simulink model "FOC"  (R2017a)
settings: Solver=VariableStepAuto  StartTime=0.0  StopTime=2.5  MaxStep=1e-4  RelTol=1e-3  EnableMultiTasking=on
values from neighbouring files (symbols this model uses):
  Ki_i = Tc/(2*Kc*Tsum)    (= 11.475)    [FOC_parameters.m]
  Ki_n = Kp_n/Ti_n    (= 1)    [FOC_parameters.m]
  Kp_i = Ki_i*Ti_i    (= 0.017)    [FOC_parameters.m]
  Kp_n = 1    [FOC_parameters.m]
  Ld = 8.5e-3    (= 0.0085)    [FOC_parameters.m]
  Lq = Ld    (= 0.0085)    [FOC_parameters.m]
  m = 1    [FOC_parameters.m]
  n_s = 1    [FOC_parameters.m]
  p = 4    [FOC_parameters.m]
  Rs = 0.0485    [FOC_parameters.m]
  Tf = 0    [FOC_parameters.m]
  Ti = 0.0027    [FOC_parameters.m]
  TL = 400    [FOC_parameters.m]
  vd = 0.0004924    [FOC_parameters.m]
libraries: powerlib x4, powerlib_meascontrol x2
settings Model: Creator=Noxma  LastModifiedBy=s181835
settings OptimizationCC: LifeSpan=inf
settings DebuggingCC: SFUnexpectedBacktrackingDiag=warning  SFNoUnconditionalDefaultTransitionDiag=warning  SFExecutionAtInitializationDiag=none
settings GRTTargetCC: TargetLangStandard=C89/C90 (ANSI)  GeneratePreprocessorConditionals=Disable all
settings ConfigComp: CovMetricSettings=dw  CovHtmlReporting=on  CovSaveCumulativeToWorkspaceVar=on  CovSaveSingleToWorkspaceVar=on  CovExternalEMLEnable=off

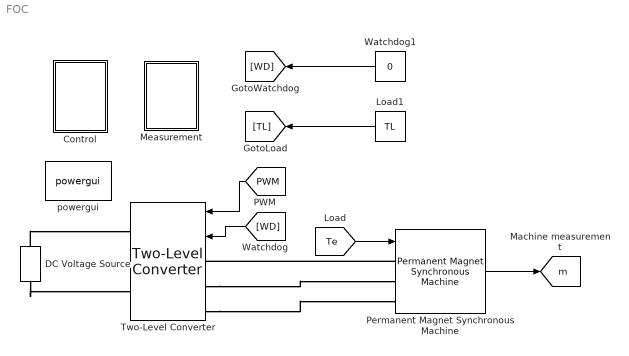
== system FOC ==
  Control : Subsystem
  DC Voltage Source : powerlib/Electrical Sources/DC Voltage Source  Amplitude=1  Measurements=None
  Load1 : Constant  Value=TL
  Measurement : Subsystem
  Permanent Magnet Synchronous Machine : powerlib/Machines/Permanent Magnet Synchronous Machine  NbPhases=3  FluxDistribution=Sinusoidal  RotorType=Salient-pole  MechanicalLoad=Torque Tm  PresetModel=No  ShowDetailedParameters=on  MeasurementBus=on  Resistance=Rs  Inductance=8.5e-3  dqInductances=[Ld,Lq]  La=0.000395  MachineConstant=Flux linkage established by magnets (V.s)  Flux=cphi  VoltageCst=86.6271  TorqueCst=0.7164  Flat=120  Mechanical=[Ti vd p Tf]  PolePairs=4  InitialConditions=[0,0, 0,0]  InitialConditions5ph=[0 0 0 0 0 0]  TsPowergui=0  TsBlock=-1  RefAngle=90 degrees behind phase A axis (modified Park)
      settings: SourceProductName=Simscape Power Systems
  Two-Level Converter : powerlib/Power Electronics/Two-Level Converter  ModelType=Switching devices  Ron=1e-3  Rs=1e6  Cs=inf  Vforward=[0,0]  Ron_Diode=1e-3  Rs_Diode=1e6  Cs_Diode=inf  Vf_Diode=1e-3  Rs_CurrentSource=inf
      settings: SourceProductName=Simscape Power Systems  SourceProductBaseCode=PS
  Watchdog1 : Constant  Value=0
  powergui : powerlib/powergui  Priority=1  SimulationMode=Continuous  SampleTime=50e-6  frequency=60  Iterations=50  frequencyindice=0  Pbase=100e6  ErrMax=1e-4  UnitsV=kV  UnitsW=MW  buscounter=0  FunctionMessages=off  echomessages=off  EnableUseOfTLC=off  CurrentSourceSwitches=off  DisableSnubberDevices=off  DisableRonSwitches=off  DisableVfSwitches=off  DisplayEquations=off  SolverType=Tustin/Backward Euler (TBE)  Interpol=off  ExternalGateDelay=off  methode=off  Ts=100  x0status=blocks  SPID=on  SwTol=0  HookPort=off  RestoreLinks=warning  ResistiveCurrentMeasurement=off  Frange=[0:2:500]  Ylog=off  Xlog=on  ShowGrid=off  save=off  variable=ZData  structure=0  ZoomFFT=off  StartTime=0.0  cycles=1  DisplayStyle=1  fundamental=60  FreqAxis=off  MaxFrequency=1000  frequencyindicesteady=1  RmsSteady=1  display=off
  tag scope: m=global
  wires:
  [PWM] -> Two-Level Converter/1
  [Te] -> Permanent Magnet Synchronous Machine/1
  Permanent Magnet Synchronous Machine/1 -> [m]
  [WD] -> Two-Level Converter/2
  Watchdog1/1 -> [WD]
  Load1/1 -> [TL]
  connections:
  Two-Level Converter/LConn3 -- Permanent Magnet Synchronous Machine/LConn3
  Two-Level Converter/LConn2 -- Permanent Magnet Synchronous Machine/LConn2
  Permanent Magnet Synchronous Machine/LConn1 -- Two-Level Converter/LConn1
  DC Voltage Source/LConn1 -- Two-Level Converter/RConn2
  DC Voltage Source/RConn1 -- Two-Level Converter/RConn1

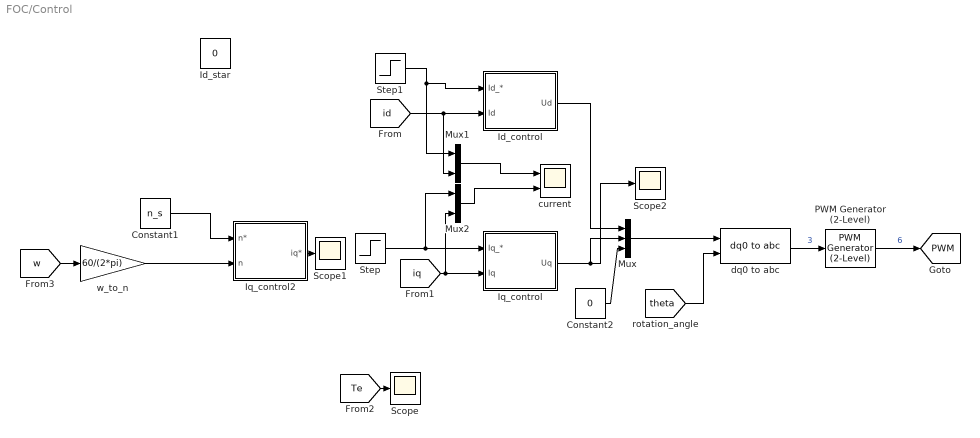
== system FOC/Control ==
  Constant1 : Constant  Value=n_s
  Constant2 : Constant  Value=0
  Id_control : Subsystem
  Id_star : Constant  Value=0
  Iq_control : Subsystem
  Iq_control2 : Subsystem
  Mux : Mux  Inputs=3
  Mux1 : Mux  Inputs=2
  Mux2 : Mux  Inputs=2
  PWM Generator (2-Level) : powerlib_meascontrol/Pulse & Signal Generators/PWM Generator (2-Level)  ModulatorType=Three-phase bridge (6 pulses)  ModulatorMode=Unsynchronized  Fc=fs  Pc=pwm_angle  nF=27  MinMax=[-m m]  SamplingTechnique=Natural  ModulatingSignals=off  m=1  Freq=f  Phase=0  Ts=0  ShowCarrierOutport=off
      settings: SourceProductName=Simscape Power Systems
  Scope : Scope
  Scope1 : Scope
  Scope2 : Scope
  Step : Step  Time=0.2  After=3  SampleTime=0
  Step1 : Step  Time=1.5  After=-1  SampleTime=0
  current : Scope  NumInputPorts=2
  dq0 to abc : powerlib_meascontrol/Transformations/dq0 to abc  Alignment=90 degrees behind phase A axis
  w_to_n : Gain  Gain=60/(2*pi)
  tag scope: PWM=global
  wires:
  PWM Generator (2-Level)/1 -> [PWM]  "6"
  [id] -> Mux1/2, Id_control/2(Id)
  [iq] -> Iq_control/2(Iq), Mux2/2
  Iq_control/1(Uq) -> Scope2/1, Mux/2
  Id_control/1(Ud) -> Mux/1
  Mux/1 -> dq0 to abc/1
  [theta] -> dq0 to abc/2
  [w] -> w_to_n/1
  w_to_n/1 -> Iq_control2/2(n)
  Constant1/1 -> Iq_control2/1(n*)
  [Te] -> Scope/1
  Constant2/1 -> Mux/3
  Step/1 -> Mux2/1, Iq_control/1(Iq_*)
  dq0 to abc/1 -> PWM Generator (2-Level)/1  "3"
  Iq_control2/1(iq*) -> Scope1/1
  Mux1/1 -> current/1
  Mux2/1 -> current/2
  Step1/1 -> Id_control/1(Id_*), Mux1/1

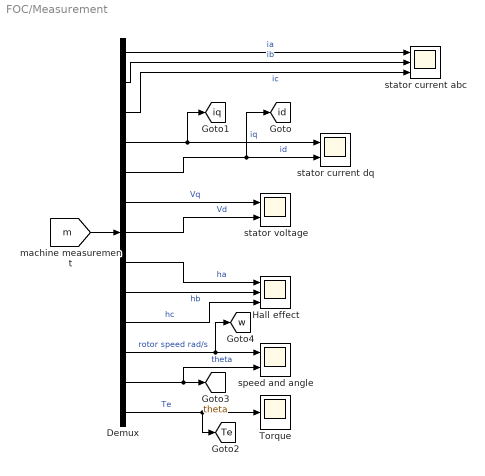
== system FOC/Measurement ==
  Demux : Demux  Outputs=13
  Hall effect : Scope  NumInputPorts=3
  Torque : Scope
  speed and angle : Scope  NumInputPorts=2
  stator current abc : Scope  NumInputPorts=3
  stator current dq : Scope  NumInputPorts=2
  stator voltage : Scope  NumInputPorts=2
  tag scope: Te=global, id=global, iq=global, theta=global, w=global
  wires:
  Demux/5 -> [id], stator current dq/2  "id"
  Demux/2 -> stator current abc/2  "ib"
  Demux/4 -> [iq], stator current dq/1  "iq"
  Demux/13 -> [Te], Torque/1  "Te"
  [m] -> Demux/1
  Demux/9 -> Hall effect/2  "hb"
  Demux/6 -> stator voltage/1  "Vq"
  Demux/11 -> [w], speed and angle/1  "rotor speed rad/s"
  Demux/12 -> [theta], speed and angle/2  "theta"
  Demux/7 -> stator voltage/2  "Vd"
  Demux/8 -> Hall effect/1  "ha"
  Demux/10 -> Hall effect/3  "hc"
  Demux/3 -> stator current abc/3  "ic"
  Demux/1 -> stator current abc/1  "ia"

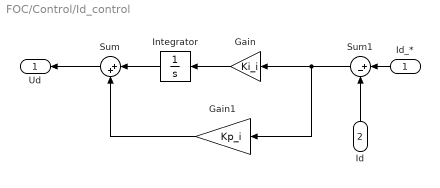
== system FOC/Control/Id_control ==
  Id_* : Inport
  Id : Inport  Port=2
  Gain : Gain  Gain=Ki_i
  Gain1 : Gain  Gain=Kp_i
  Integrator : Integrator
  Sum : Sum  Inputs=|++
  Sum1 : Sum  Inputs=|+-
  Ud : Outport
  wires:
  Sum/1 -> Ud/1
  Integrator/1 -> Sum/1
  Gain1/1 -> Sum/2
  Gain/1 -> Integrator/1
  Sum1/1 -> Gain1/1, Gain/1
  Id_*/1 -> Sum1/1
  Id/1 -> Sum1/2

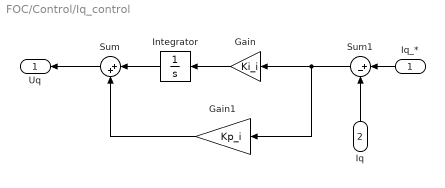
== system FOC/Control/Iq_control ==
  Iq_* : Inport
  Iq : Inport  Port=2
  Gain : Gain  Gain=Ki_i
  Gain1 : Gain  Gain=Kp_i
  Integrator : Integrator
  Sum : Sum  Inputs=|++
  Sum1 : Sum  Inputs=|+-
  Uq : Outport
  wires:
  Sum/1 -> Uq/1
  Integrator/1 -> Sum/1
  Gain1/1 -> Sum/2
  Gain/1 -> Integrator/1
  Sum1/1 -> Gain1/1, Gain/1
  Iq_*/1 -> Sum1/1
  Iq/1 -> Sum1/2

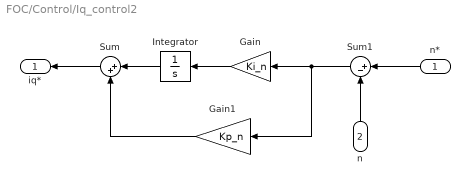
== system FOC/Control/Iq_control2 ==
  n* : Inport
  n : Inport  Port=2
  Gain : Gain  Gain=Ki_n
  Gain1 : Gain  Gain=Kp_n
  Integrator : Integrator
  Sum : Sum  Inputs=|++
  Sum1 : Sum  Inputs=|+-
  iq* : Outport
  wires:
  Sum/1 -> iq*/1
  Integrator/1 -> Sum/1
  Gain1/1 -> Sum/2
  Gain/1 -> Integrator/1
  Sum1/1 -> Gain1/1, Gain/1
  n/1 -> Sum1/2
  n*/1 -> Sum1/1
